simulink model "crazyflie"  (R2022b)
settings: Solver=FixedStepAuto  StartTime=0.0  StopTime=160  FixedStep=0.001  RelTol=1e-3
values from neighbouring files (symbols this model uses):
  g = 9.81    [ModelForCrazyfile.m]    (also in linearization.m; params.m)
  L = dlqr(A_d,B_d,Q_x,Q_u)    [ModelForCrazyfile.m]
settings Model: PauseTimes=7  Creator=Zrean  LastModifiedBy=liqui
settings SolverCC: AlgebraicLoopSolver=TrustRegion
settings DataIOCC: ReturnWorkspaceOutputs=off
settings OptimizationCC: DefaultParameterBehavior=Inlined  UseDivisionForNetSlopeComputation=on  UseFloatMulNetSlope=on  UseSpecifiedMinMax=on  InlineInvariantSignals=on  PassReuseOutputArgsAs=Individual arguments  ZeroExternalMemoryAtStartup=off  ZeroInternalMemoryAtStartup=off  NoFixptDivByZeroProtection=on  EfficientFloat2IntCast=on  LifeSpan=1  EfficientTunableParamExpr=on
settings DebuggingCC: AlgebraicLoopMsg=error  ParameterTunabilityLossMsg=error  UnconnectedInputMsg=warning  UnconnectedOutputMsg=warning  UnconnectedLineMsg=warning  SFMachineParentedDataDiag=warning  ArithmeticOperatorsInVariantConditions=warning
settings HardwareCC: ProdBitPerPointer=32  ProdBitPerSizeT=32  ProdBitPerPtrDiffT=32  ProdLargestAtomicInteger=Long  ProdLargestAtomicFloat=Double  ProdWordSize=32  ProdHWDeviceType=ARM Compatible->ARM Cortex
settings ModelReferenceCC: EnableRefExpFcnMdlSchedulingChecks=on
settings SFSimCC: SimUseLocalCustomCode=off  MATLABDynamicMemAlloc=off  CustomCodeUndefinedFunction=UseInterfaceOnly
settings RTWCC: Description=Embedded Coder  SystemTargetFile=ert.tlc  GenCodeOnly=on  TemplateMakefile=ert_default_tmf  GenerateReport=on  RTWUseLocalCustomCode=off  BuildConfiguration=Faster Runs  IncludeHyperlinkInReport=on  LaunchReport=on  GenerateTraceInfo=on  GenerateTraceReport=on  GenerateTraceReportSl=on  GenerateTraceReportSf=on  GenerateTraceReportEml=on  GenerateCodeMetricsReport=on
settings CodeAppCC: ForceParamTrailComments=on  IgnoreCustomStorageClasses=off  OperatorAnnotations=on  SimulinkDataObjDesc=on  SFDataObjDesc=on  MATLABFcnDesc=on  InsertBlockDesc=on  StateflowObjectComments=on  MATLABSourceComments=on
settings ERTTargetCC: TargetLangStandard=C99 (ISO)  MultiwordLength=2048  CombineSignalStateStructs=on  SuppressErrorStatus=on  SupportAbsoluteTime=off  SupportNonFinite=off  SupportComplex=off  InlinedParameterPlacement=NonHierarchical  ERTCustomFileTemplate=crazyflie_wrapper.tlc  ERTFilePackagingFormat=CompactWithDataFile
settings SimscapeCC: SimscapeNormalizeSystem=off

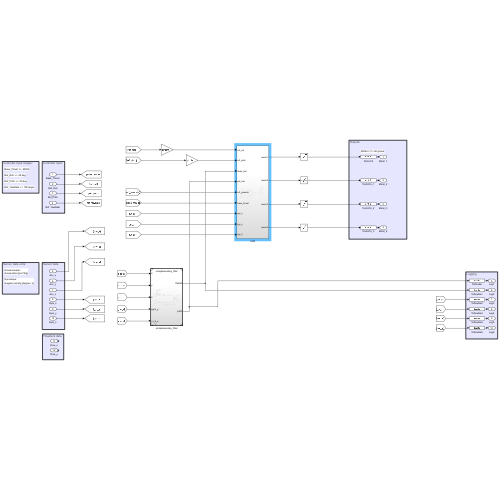
[thumbnail: Simulink's stored preview of the top-level diagram]
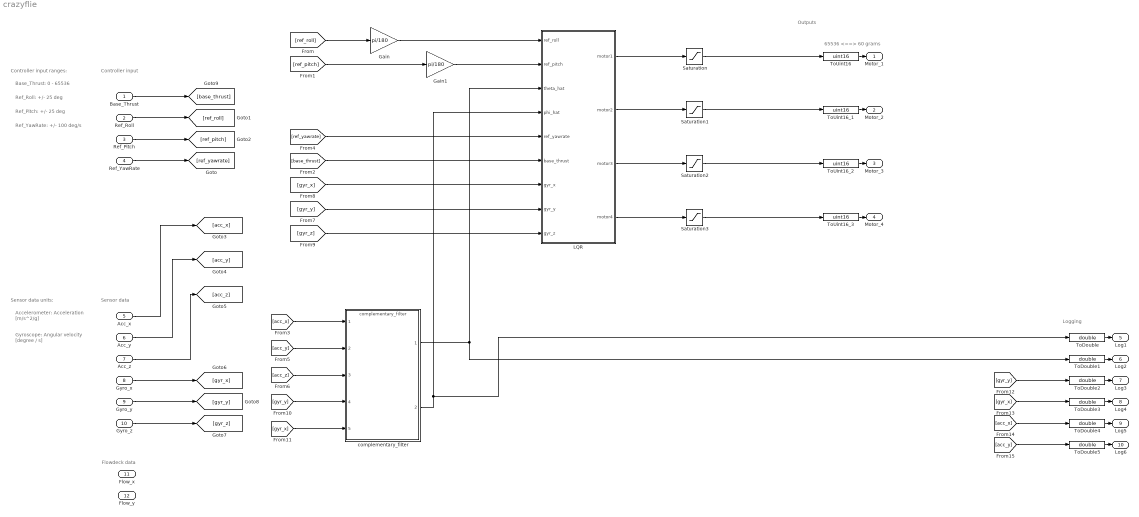
== system crazyflie ==
  note: 65536 <==> 60 grams
  note: Logging
  note: Outputs
  note: Sensor data
  note: Controller input
  note: Ref_Roll: +/- 25 deg
  note: Base_Thrust: 0 - 65536
  note: Ref_Pitch: +/- 25 deg
  note: Ref_YawRate: +/- 100 deg/s
  note: Controller input ranges:
  note: Gyroscope:
      | Angular velocity [degree / s]
  note: Accelerometer:
      | Acceleration [m/s^2/g]
  note: Sensor data units:
  note: Flowdeck data
  Base_Thrust : Inport  OutDataTypeStr=double
  Ref_Roll : Inport  Port=2  OutDataTypeStr=double
  Ref_Pitch : Inport  Port=3  OutDataTypeStr=double
  Ref_YawRate : Inport  Port=4  OutDataTypeStr=double
  Acc_x : Inport  Port=5  OutDataTypeStr=double  PortDimensions=1
  Acc_y : Inport  Port=6  OutDataTypeStr=double  PortDimensions=1
  Acc_z : Inport  Port=7  OutDataTypeStr=double  PortDimensions=1
  Gyro_x : Inport  Port=8  OutDataTypeStr=double  PortDimensions=1
  Gyro_y : Inport  Port=9  OutDataTypeStr=double  PortDimensions=1
  Gyro_z : Inport  Port=10  OutDataTypeStr=double  PortDimensions=1
  Flow_x : Inport  Port=11  OutDataTypeStr=int16  PortDimensions=1
  Flow_y : Inport  Port=12  OutDataTypeStr=int16  PortDimensions=1
  Gain : Gain  Gain=pi/180
  Gain1 : Gain  Gain=pi/180
  LQR : Subsystem
  Saturation{,1..3} (4 alike) : Saturate  UpperLimit=65536  LowerLimit=0
  ToDouble{,1..5} (6 alike) : DataTypeConversion  OutDataTypeStr=double  RndMeth=Floor
  ToUint16 : DataTypeConversion  OutDataTypeStr=uint16  RndMeth=Floor
  ToUint16_1 : DataTypeConversion  OutDataTypeStr=uint16  RndMeth=Floor
  ToUint16_2 : DataTypeConversion  OutDataTypeStr=uint16  RndMeth=Floor
  ToUint16_3 : DataTypeConversion  OutDataTypeStr=uint16  RndMeth=Floor
  complementary_filter : ModelReference  ModelNameDialog=complementary_filter.slx  SimulationMode=Normal  ModelReferenceVersion=1.7
  Motor_1 : Outport  OutDataTypeStr=uint16  VectorParamsAs1DForOutWhenUnconnected=off  LockScale=on
  Motor_2 : Outport  Port=2  OutDataTypeStr=uint16  VectorParamsAs1DForOutWhenUnconnected=off  LockScale=on
  Motor_3 : Outport  Port=3  OutDataTypeStr=uint16  VectorParamsAs1DForOutWhenUnconnected=off  LockScale=on
  Motor_4 : Outport  Port=4  OutDataTypeStr=uint16  VectorParamsAs1DForOutWhenUnconnected=off  LockScale=on
  Log1 : Outport  Port=5  OutDataTypeStr=double  VectorParamsAs1DForOutWhenUnconnected=off
  Log2 : Outport  Port=6  OutDataTypeStr=double  VectorParamsAs1DForOutWhenUnconnected=off
  Log3 : Outport  Port=7  OutDataTypeStr=double  VectorParamsAs1DForOutWhenUnconnected=off
  Log4 : Outport  Port=8  OutDataTypeStr=double  VectorParamsAs1DForOutWhenUnconnected=off
  Log5 : Outport  Port=9  OutDataTypeStr=double  VectorParamsAs1DForOutWhenUnconnected=off
  Log6 : Outport  Port=10  OutDataTypeStr=double  VectorParamsAs1DForOutWhenUnconnected=off
  wires:
  ToUint16/1 -> Motor_1/1
  ToUint16_1/1 -> Motor_2/1
  ToUint16_2/1 -> Motor_3/1
  ToUint16_3/1 -> Motor_4/1
  ToDouble/1 -> Log1/1
  ToDouble1/1 -> Log2/1
  ToDouble2/1 -> Log3/1
  ToDouble3/1 -> Log4/1
  ToDouble4/1 -> Log5/1
  ToDouble5/1 -> Log6/1
  Acc_x/1 -> [acc_x]
  Acc_y/1 -> [acc_y]
  Acc_z/1 -> [acc_z]
  Gyro_x/1 -> [gyr_x]
  Gyro_y/1 -> [gyr_y]
  Ref_YawRate/1 -> [ref_yawrate]
  Ref_Pitch/1 -> [ref_pitch]
  Ref_Roll/1 -> [ref_roll]
  Gyro_z/1 -> [gyr_z]
  [ref_pitch] -> Gain1/1
  [ref_yawrate] -> LQR/5(ref_yawrate)
  [gyr_x] -> LQR/7(gyr_x)
  [gyr_y] -> LQR/8(gyr_y)
  [gyr_z] -> LQR/9(gyr_z)
  Base_Thrust/1 -> [base_thrust]
  [base_thrust] -> LQR/6(base_thrust)
  LQR/1(motor1) -> Saturation/1
  Saturation/1 -> ToUint16/1
  LQR/2(motor2) -> Saturation1/1
  Saturation1/1 -> ToUint16_1/1
  LQR/3(motor3) -> Saturation2/1
  Saturation2/1 -> ToUint16_2/1
  Saturation3/1 -> ToUint16_3/1
  LQR/4(motor4) -> Saturation3/1
  [acc_x] -> complementary_filter/1
  complementary_filter/1 -> LQR/3(theta_hat), ToDouble1/1
  complementary_filter/2 -> ToDouble/1, LQR/4(phi_hat)
  [acc_y] -> complementary_filter/2
  [gyr_x] -> complementary_filter/5
  [acc_z] -> complementary_filter/3
  [gyr_y] -> ToDouble2/1
  [gyr_x] -> ToDouble3/1
  [acc_x] -> ToDouble4/1
  [acc_y] -> ToDouble5/1
  [gyr_y] -> complementary_filter/4
  Gain/1 -> LQR/1(ref_roll)
  Gain1/1 -> LQR/2(ref_pitch)
  [ref_roll] -> Gain/1

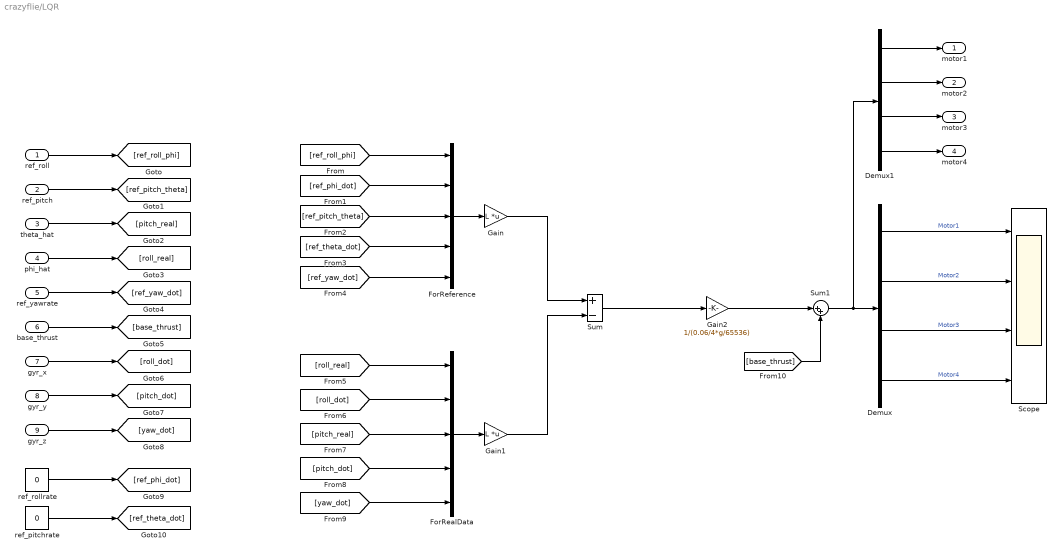
== system crazyflie/LQR ==
  ref_roll : Inport
  ref_pitch : Inport  Port=2
  theta_hat : Inport  Port=3
  phi_hat : Inport  Port=4
  ref_yawrate : Inport  Port=5
  base_thrust : Inport  Port=6
  gyr_x : Inport  Port=7
  gyr_y : Inport  Port=8
  gyr_z : Inport  Port=9
  Demux : Demux
  Demux1 : Demux
  ForRealData : Mux  Inputs=5
  ForReference : Mux  Inputs=5
  Gain : Gain  Gain=L  Multiplication=Matrix(K*u)
  Gain1 : Gain  Gain=L  Multiplication=Matrix(K*u)
  Gain2 : Gain  Gain=1/(0.06/4*g/65536)
  Scope : Scope  NumInputPorts=4
  Sum : Sum  Inputs=+-
  Sum1 : Sum  Inputs=|++
  ref_pitchrate : Constant  Value=0
  ref_rollrate : Constant  Value=0
  motor1 : Outport
  motor2 : Outport  Port=2
  motor3 : Outport  Port=3
  motor4 : Outport  Port=4
  wires:
  ref_roll/1 -> [ref_roll_phi]
  ref_pitch/1 -> [ref_pitch_theta]
  theta_hat/1 -> [pitch_real]
  phi_hat/1 -> [roll_real]
  ref_yawrate/1 -> [ref_yaw_dot]
  base_thrust/1 -> [base_thrust]
  [ref_roll_phi] -> ForReference/1
  ref_rollrate/1 -> [ref_phi_dot]
  ref_pitchrate/1 -> [ref_theta_dot]
  gyr_x/1 -> [roll_dot]
  gyr_y/1 -> [pitch_dot]
  gyr_z/1 -> [yaw_dot]
  [ref_phi_dot] -> ForReference/2
  [ref_pitch_theta] -> ForReference/3
  [ref_theta_dot] -> ForReference/4
  [ref_yaw_dot] -> ForReference/5
  [roll_real] -> ForRealData/1
  [pitch_real] -> ForRealData/3
  [roll_dot] -> ForRealData/2
  [pitch_dot] -> ForRealData/4
  [yaw_dot] -> ForRealData/5
  ForReference/1 -> Gain/1
  ForRealData/1 -> Gain1/1
  Demux1/1 -> motor1/1
  Demux1/2 -> motor2/1
  Demux1/3 -> motor3/1
  Demux1/4 -> motor4/1
  Demux/1 -> Scope/1  "Motor1"
  Demux/2 -> Scope/2  "Motor2"
  Demux/3 -> Scope/3  "Motor3"
  Demux/4 -> Scope/4  "Motor4"
  Sum/1 -> Gain2/1
  Sum1/1 -> Demux1/1, Demux/1
  [base_thrust] -> Sum1/2
  Gain1/1 -> Sum/2
  Gain2/1 -> Sum1/1
  Gain/1 -> Sum/1
